simulink model "Roombaavancet_newnewnewnew"  (R2018b)
settings: Solver=FixedStepDiscrete  StartTime=0.0  StopTime=inf  FixedStep=0.1  RelTol=1e-3
InitFcn:
  | iRobotControl_switchyard('setup_localPCclock');iRobotControl_switchyard('setup_StarGazer_landmark_offset_table')
undefined symbols (not defined in the file or in its folder): iRobotControl_switchyard, none, Rec, SDTV, videoinput
libraries: visiontransforms x2, visionconversions x1, visiontextngfix x1, visionanalysis x1, visionstatistics x1, imaqlib x1, realtime_pacer_lib x1, visionsinks x1
CloseFcn:
  | iRobotControl_switchyard close_iRobotControl
settings Model: Creator=sksu  LastModifiedBy=chada
settings SolverCC: PositivePriorityOrder=on
settings DataIOCC: LimitDataPoints=on  SaveFormat=Array  SignalLoggingSaveFormat=ModelDataLogs
settings OptimizationCC: EnhancedBackFolding=on  PassReuseOutputArgsAs=Individual arguments  ExpressionDepthLimit=2147483647  MaxStackSize=64  OptimizeBlockOrder=speed  DifferentSizesBufferReuse=on  OptimizationCustomize=off
settings DebuggingCC: UnderspecifiedInitializationDetection=Classic  MergeDetectMultiDrivingBlocksExec=none  SolverPrmCheckMsg=warning  ParameterTunabilityLossMsg=error  FcnCallInpInsideContextMsg=warning  AllowSymbolicDim=off  StateNameClashWarn=warning  SFUnexpectedBacktrackingDiag=warning  SFNoUnconditionalDefaultTransitionDiag=warning  SFExecutionAtInitializationDiag=none
settings HardwareCC: ProdBitPerPointer=32  ProdBitPerSizeT=32  ProdBitPerPtrDiffT=32  ProdLargestAtomicInteger=Long  ProdLargestAtomicFloat=Double  ProdWordSize=32  ProdHWDeviceType=ARM Compatible->ARM Cortex
settings ModelReferenceCC: PropagateSignalLabelsOutOfModel=off
settings SFSimCC: SimUseLocalCustomCode=off  MATLABDynamicMemAlloc=off
settings RTWCC: SystemTargetFile=ert.tlc  HardwareBoard=Raspberry Pi  TLCOptions="-aInlineSetEventsForThisBaseRateFcn=TLC_FALSE -aSuppressMultiTaskScheduler=TLC_FALSE  -aRateBasedStepFcn=0"  TemplateMakefile=ert_default_tmf  GenerateReport=on  RTWUseLocalCustomCode=off  Toolchain=GNU GCC Raspberry Pi  BuildConfiguration=Faster Runs  IncludeHyperlinkInReport=on  LaunchReport=on  GenerateTraceInfo=on  GenerateTraceReport=on  GenerateTraceReportSl=on  GenerateTraceReportSf=on  GenerateTraceReportEml=on
settings CodeAppCC: ForceParamTrailComments=on  IgnoreCustomStorageClasses=off  OperatorAnnotations=on  SimulinkDataObjDesc=on  SFDataObjDesc=on  InsertBlockDesc=on
settings ERTTargetCC: SupportVariableSizeSignals=on
settings ConfigComp: CovMetricSettings=dw  CovHtmlReporting=on  CovSaveCumulativeToWorkspaceVar=on  CovSaveSingleToWorkspaceVar=on  CovExternalEMLEnable=off

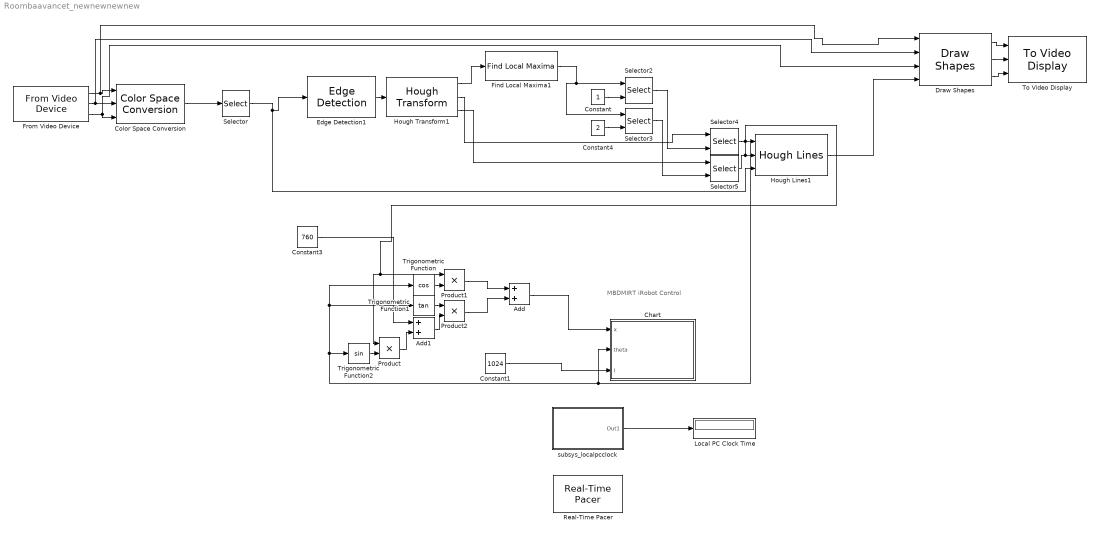
== system Roombaavancet_newnewnewnew ==
  note: MBDMIRT iRobot Control
  Add : Sum
  Add1 : Sum
  Chart : Stateflow chart  TreatAsAtomicUnit=on
  Color Space Conversion : visionconversions/Color Space  Conversion  conversion=Obsolete  conversionActive=R'G'B' to intensity  wp_str=D65  rec=Rec. 601 (SDTV)  sys=1125/60/2:1  imagePorts=Separate color signals
      settings: SourceProductName=Computer Vision System Toolbox
  Constant : Constant
  Constant1 : Constant  Value=1024
  Constant3 : Constant  Value=760
  Constant4 : Constant  Value=2
  Draw Shapes : visiontextngfix/Draw Shapes  shape=Lines  fill=off  lineWidth=10  fillClrSource=Specify via dialog  display=User-specified value  intensity=200  color=[000 000 255]  opacity=0.6  viewport=Entire image  antialiasing=off  inType=Obsolete  imagePorts=Separate color signals  prodOutputMode=Binary point scaling  prodOutputWordLength=32  prodOutputFracLength=14  memoryMode=Specify word length  memoryWordLength=16  memoryFracLength=14  roundingMode=Floor  overflowMode=off
      settings: SourceProductName=Computer Vision System Toolbox
  Edge Detection1 : visionanalysis/Edge Detection  method=Sobel  outputType=Binary image  userDefinedThreshold=off  thresholdSource=Input port  threshold=20  thresholdTuning=4  edgeThinning=off  threshold_canny=[0.25 0.60]  autoPercent=70  sigma=1  roundingMode=Floor  overflowMode=off  prodOutputMode=Binary point scaling  prodOutputWordLength=32  prodOutputFracLength=8  prodOutputSlope=2^-8  accumSlope=2^-8  outputSlope=2^-4
      settings: SourceProductName=Computer Vision System Toolbox  SourceProductBaseCode=VP
  Find Local Maxima1 : visionstatistics/Find Local Maxima  num_peaks=1  nhood_size=[801 201]  src_thresh=Obsolete9b  src_thresh_inuse=Specify via dialog  threshold=10  inputIsHough=on  dt_peak=uint32  isOutVarDim=on  dt_count=uint32
      settings: SourceProductName=Computer Vision System Toolbox  SourceProductBaseCode=VP
  From Video Device : imaqlib/From Video Device  DeviceMenu=(none)  Device=winvideo 1 (Webcam C170)  ObjConstructor=videoinput('winvideo', 1)  VideoFormatMenu=(none)  VideoFormat=MJPG_1024x768  VideoSource=input1  ROIPosition=[0 0 768 1024]  EnableHWTrigger=off  TriggerConfiguration=none/none  SampleTime=0.1  OutputPortsMode=Separate color signals  DataType=single  CanDoHWTrigger=no  ReturnedColorSpace=rgb  BlockHandle=146.0004  ROIWidth=1024  ROIHeight=768  ROIColumn=0  ROIRow=0  EngXMLPath=C:\Program Files\MATLAB\R2018b\toolbox\imaq\imaq\private  DevXMLPath=C:\ProgramData\MATLAB\SupportPackages\R2018b\toolbox\imaq\supportpackages\genericvideo\adaptor\win64  EngLibPath=C:\Program Files\MATLAB\R2018b\toolbox\imaq\imaqblks\imaqmex\win64  ColorSpace=rgb  BayerSensorAlignment=grbg
      settings: SourceProductName=Image Acquisition Toolbox
  Hough Lines1 : visiontransforms/Hough Lines  sineCompMethod=Trigonometric function  thetaRes=pi/180  firstCoeffMode=Specify word length  firstCoeffWordLength=16  firstCoeffFracLength=15  prodOutputMode=Binary point scaling  prodOutputWordLength=32  prodOutputFracLength=16  roundingMode=Nearest  overflowMode=on
      settings: SourceProductName=Computer Vision System Toolbox  SourceProductBaseCode=VP
  Hough Transform1 : visiontransforms/Hough Transform  theta_res=pi/360  rho_res=1  out_theta_rho=on  outdtmode=double  roundingMode=Nearest  overflowMode=on  firstCoeffMode=Binary point scaling  firstCoeffWordLength=16  firstCoeffFracLength=14  firstCoeffSlope=2^-14  secondCoeffMode=Binary point scaling  secondCoeffWordLength=32  secondCoeffFracLength=16  secondCoeffSlope=2^-16  prodOutputMode=Binary point scaling  prodOutputWordLength=32  prodOutputFracLength=20  prodOutputSlope=2^-20  accumMode=Binary point scaling  accumWordLength=32  accumFracLength=20  accumSlope=2^-20  outputMode=Binary point scaling  outputWordLength=16  outputFracLength=0  outputSlope=2^0  memoryMode=Binary point scaling  memoryWordLength=32  memoryFracLength=16  memorySlope=2^-16
      settings: SourceProductName=Computer Vision System Toolbox  SourceProductBaseCode=VP
  Local PC Clock Time : Display
  Product : Product
  Product1 : Product
  Product2 : Product
  Real-Time Pacer : realtime_pacer_lib/Real-Time Pacer  simTimePerRealTime=1000
  Selector : Selector  NumberOfDimensions=2  InputPortWidth=3  IndexOptions=Starting index (dialog),Select all  Indices=[1],1  OutputSizes=[760],1
  Selector2 : Selector  InputPortWidth=2  IndexOptions=Index vector (port)  Indices=1  OutputSizes=1
  Selector3 : Selector  InputPortWidth=2  IndexOptions=Index vector (port)  Indices=0  OutputSizes=1
  Selector4 : Selector  InputPortWidth=360  IndexOptions=Index vector (port)  Indices=[1 3]  OutputSizes=1
  Selector5 : Selector  InputPortWidth=2549  IndexOptions=Index vector (port)  Indices=[1 3]  OutputSizes=1
  To Video Display : visionsinks/To Video Display  windowSizeMode=Normal  openAtMdlStart=on  fullScreen=off  videoWindowX=0  videoWindowY=22  saveWindowSize=off  videoWindowWidth=1440  videoWindowHeight=838  inputColorFormat=RGB  inputType=Obsolete  imagePorts=Separate color signals  OutputDevice=On-screen video monitor  dataOrg=Column-major  isWindowOpen=off
      settings: SourceProductName=Computer Vision System Toolbox
  Trigonometric Function : Trigonometry  Operator=cos
  Trigonometric Function1 : Trigonometry  Operator=tan
  Trigonometric Function2 : Trigonometry
  subsys_localpcclock : Subsystem
      mask Display: fprintf('Elapsed Local PC\nClock')
  wires:
  subsys_localpcclock/1(Out1) -> Local PC Clock Time/1
  Trigonometric Function/1 -> Product1/2
  Product1/1 -> Add/1
  Product2/1 -> Add/2
  Trigonometric Function1/1 -> Product2/1
  Add1/1 -> Product2/2
  Product/1 -> Add1/2
  Trigonometric Function2/1 -> Product/2
  Selector4/1 -> Chart/2(theta), Trigonometric Function1/1, Trigonometric Function/1, Trigonometric Function2/1, Hough Lines1/1
  Selector5/1 -> Product/1, Product1/1, Hough Lines1/2
  Constant3/1 -> Add1/1
  Constant4/1 -> Selector3/2
  Hough Transform1/3 -> Selector5/1
  Hough Transform1/2 -> Selector4/1
  Selector2/1 -> Selector4/2
  Selector3/1 -> Selector5/2
  Edge Detection1/1 -> Hough Transform1/1
  Constant/1 -> Selector2/2
  Find Local Maxima1/1 -> Selector3/1, Selector2/1
  Hough Transform1/1 -> Find Local Maxima1/1
  From Video Device/2 -> Color Space Conversion/2, Draw Shapes/2
  From Video Device/1 -> Draw Shapes/1, Color Space Conversion/1
  From Video Device/3 -> Color Space Conversion/3, Draw Shapes/3
  Hough Lines1/1 -> Draw Shapes/4
  Draw Shapes/2 -> To Video Display/2
  Draw Shapes/1 -> To Video Display/1
  Draw Shapes/3 -> To Video Display/3
  Color Space Conversion/1 -> Selector/1
  Selector/1 -> Hough Lines1/3, Edge Detection1/1
  Add/1 -> Chart/1(x)
  Constant1/1 -> Chart/3(l)

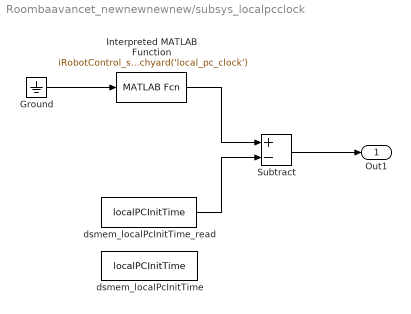
== system Roombaavancet_newnewnewnew/subsys_localpcclock ==
  Ground : Ground
  Interpreted MATLAB Function : MATLABFcn  MATLABFcn=iRobotControl_switchyard('local_pc_clock')  OutputSignalType=real
  Subtract : Sum  Inputs=+-
  dsmem_localPcInitTime : DataStoreMemory  DataStoreName=localPCInitTime  WriteAfterWriteMsg=warning  WriteAfterReadMsg=warning  InitialValue=2390464.087  ShowAdditionalParam=off  OutDataTypeStr=double
  dsmem_localPcInitTime_read : DataStoreRead  DataStoreName=localPCInitTime  SampleTime=1
  Out1 : Outport
  wires:
  Ground/1 -> Interpreted MATLAB Function/1
  Interpreted MATLAB Function/1 -> Subtract/1
  dsmem_localPcInitTime_read/1 -> Subtract/2
  Subtract/1 -> Out1/1

== stateflow chart Roombaavancet_newnewnewnew/Chart ==
  settings: updateMethod=DISCRETE  sampleTime=1
  state AngleR = AngleSensorRoomba(serObjNum) [function]
    (default) -> (junction 640) : { AngleR = ml('AngleSensorRoomba(iRobot_%d)', serObjNum); }
  state clk = LocalPCClock [function]
    (default) -> (junction 1924) : {clk = ml.iRobotControl_switchyard('local_pc_clock');}
  state state = CliffRightSensorRoomba(serObjNum) [function]
    (default) -> (junction 756) : { state = ml('CliffRightSensorRoomba(iRobot_%d)', serObjNum); }
  state [Charge, Capacity, Percent] = BatteryChargeReaderRoomba(serObjNum) [function]
    (default) -> (junction 665) : {
        | /* Reset container for battery status */
        | ml('iRobot_%d_BattCharSensor(1:3)=0;', serObjNum);
        |
        | /* Read battery status */
        | ml('[iRobot_%d_BattCharSensor(1), iRobot_%d_BattCharSensor(2), iRobot_%d_BattCharSensor(3)]=BatteryChargeReaderRoomba(iRobot_%d);',...
        |       serObjNum, serObjNum, serObjNum, serObjNum);
        |
        |
        | BattCharSensor=ml('iRobot_%d_BattCharSensor', serObjNum);
        |
        | Charge=BattCharSensor[0];
        | Capacity=BattCharSensor[1];
        | Percent=BattCharSensor[2];
        | }
  state strg = CliffRightSignalStrengthRoomba(serObjNum) [function]
    (default) -> (junction 761) : { strg = ml('CliffRightSignalStrengthRoomba(iRobot_%d)', serObjNum); }
  state BeepRoomba(serObjNum) [function]
    (default) -> (junction 686) : { ml('BeepRoomba(iRobot_%d)', serObjNum); }
  state iRobot_Test
    state INIT
      en: irobotID=1;
      serObjNum=RoombaInit(irobotID)
    state DEPLACEMENT
      du:
      [Dock, Clean] = ButtonsSensorRoomba(serObjNum);
      state STOP
        en: SetFwdVelAngVelCreate(serObjNum, 0, 0);
        SetLEDsRoomba(serObjNum, 0, 10, 100);
        SetBrushRoomba(serObjNum, 0);
      state Fwd_Bwd
        state Robot_avance_vitesseConstante
          en:
          SetFwdVelAngVelCreate(serObjNum, 0.05, 0);
          seenClk=LocalPCClock();
          du:
          currClk=LocalPCClock();
        state corrige
          en:
          SetFwdVelAngVelCreate(serObjNum,0.05,- 0.1*(theta)/(abs(theta)));
        (default) -> Robot_avance_vitesseConstante
        corrige -> Robot_avance_vitesseConstante : [abs(x-(l/2))<1 && abs(theta)<0.2]
        Robot_avance_vitesseConstante -> corrige : [abs(x-(l/2))>1 || abs(theta)>0.2]
      (default) -> STOP
      Fwd_Bwd -> STOP : [Dock]
      STOP -> Fwd_Bwd : [Clean]
    note: ?
    (default) -> INIT
    INIT -> DEPLACEMENT
  state [BumpRight, BumpLeft, WheDropRight, WheDropLeft, ... [function]
    WheDropCaster, BumpFront] = BumpsWheelDropsSensorsRoomba(serObjNum)
    (default) -> (junction 455) : {
        | /* Reset container for bump and wheel sensors */
        | ml('iRobot_%d_BmpWhlSensor(1:6)=0;', serObjNum);
        |
        | /* Read bump and wheel sensors */
        | ml('[iRobot_%d_BmpWhlSensor(1), iRobot_%d_BmpWhlSensor(2), iRobot_%d_BmpWhlSensor(3), iRobot_%d_BmpWhlSensor(4), iRobot_%d_BmpWhlSensor(5), iRobot_%d_BmpWhlSensor(6)]=BumpsWheelDropsSensorsRoomba(iRobot_%d);',...
        |       serObjNum, serObjNum, serObjNum, serObjNum, serObjNum, serObjNum, serObjNum);
        |
        |
        | BmpWhlSensor = ml('iRobot_%d_BmpWhlSensor', serObjNum);
        |
        | BumpRight=BmpWhlSensor[0];
        | BumpLeft=BmpWhlSensor[1];
        | WheDropRight=BmpWhlSensor[2];
        | WheDropLeft=BmpWhlSensor[3];
        | WheDropCaster=BmpWhlSensor[4];
        | BumpFront=BmpWhlSensor[5];
        | }
  state Current = CurrentTesterRoomba(serObjNum) [function]
    (default) -> (junction 766) : { Current = ml('CurrentTesterRoomba(iRobot_%d)', serObjNum); }
  state [ButtonAdv, ButtonPlay] = ButtonsSensorRoomba(serObjNum) [function]
    (default) -> (junction 694) : {
        | /* Reset container for buttons seonsor */
        | ml('iRobot_%d_ButtSensor(1:2)=0;', serObjNum);
        |
        | /* Read battery status */
        | ml('[iRobot_%d_ButtSensor(1), iRobot_%d_ButtSensor(2)]=ButtonsSensorRoomba(iRobot_%d);',...
        |       serObjNum, serObjNum, serObjNum);
        |
        |
        | ButtSensor=ml('iRobot_%d_ButtSensor', serObjNum);
        |
        | ButtonAdv=ButtSensor[0];
        | ButtonPlay=ButtSensor[1];
        | }
  state Distance = DistanceSensorRoomba(serObjNum) [function]
    (default) -> (junction 801) : { Distance = ml('DistanceSensorRoomba(iRobot_%d)', serObjNum); }
  state state = CliffFrontLeftSensorRoomba(serObjNum) [function]
    (default) -> (junction 718) : { state = ml('CliffFrontLeftSensorRoomba(iRobot_%d)', serObjNum); }
  state serObjNum = RoombaInit(irobotID) [function]
    (default) -> (junction 574) : /* Check if expected variable exists*/
        | { flag_exist=ml('exist(''iRobot_%d'',''var'')', irobotID); }
    (junction 574) -> (junction 575) [order 1] : [ flag_exist==true ]
    (junction 575) -> (junction 580) : /* Check if the expected variable is a serial object */
        | { flag_serport=ml('isa(iRobot_%d, ''serial'')', irobotID); }
    (junction 574) -> (junction 578) [order 2]
    (junction 580) -> (junction 576) [order 1] : [ flag_serport==true ]
    (junction 580) -> (junction 577) [order 2]
    (junction 576) -> (junction 581) : { serObjNum=irobotID; }
    (junction 577) -> (junction 578)
    (junction 578) -> (junction 2272) : { ml.error('iRobot_%d is not initialized.', irobotID); }
  state strg = CliffFrontLeftSignalStrengthRoomba(serObjNum) [function]
    (default) -> (junction 729) : { strg = ml('CliffFrontLeftSignalStrengthRoomba(iRobot_%d)', serObjNum); }
  state SetDriveWheelsCreate(serObjNum, rightWheelVel, leftWheelVel) [function]
    (default) -> (junction 809) : { ml('SetDriveWheelsCreate(iRobot_%d, %f, %f)', serObjNum, rightWheelVel, leftWheelVel); }
  state state = CliffFrontRightSensorRoomba(serObjNum) [function]
    (default) -> (junction 736) : { state = ml('CliffFrontRightSensorRoomba(iRobot_%d)', serObjNum); }
  state SetFwdVelAngVelCreate(serObjNum, FwdVel, AngVel) [function]
    (default) -> (junction 65) : { ml('SetFwdVelAngVelCreate(iRobot_%d, %f, %f)', serObjNum, FwdVel, AngVel); }
  state SetBrushRoomba(serObjNum, Brushes) [function]
    (default) -> (junction 3475) : { ml('SetBrushRoomba(iRobot_%d, %f)', serObjNum, Brushes); }
  state SetFwdVelRadiusRoomba(serObjNum, FwdVel, Radius) [function]
    (default) -> (junction 816) : { ml('SetFwdVelRadiusRoomba(iRobot_%d, %f, %f)', serObjNum, FwdVel, Radius); }
  state strg = CliffFrontRightSignalStrengthRoomba(serObjNum) [function]
    (default) -> (junction 741) : { strg = ml('CliffFrontRightSignalStrengthRoomba(iRobot_%d)', serObjNum); }
  state SetLCDRoomba(serObjNum, D3,D2,D1,D0) [function]
    (default) -> (junction 3466) : { ml('SetLCDRoomba(iRobot_%d, %f, %f, %f, %f)', serObjNum, D3, D2, D1, D0); }
  state state = CliffLeftSensorRoomba(serObjNum) [function]
    (default) -> (junction 746) : { state = ml('CliffLeftSensorRoomba(iRobot_%d)', serObjNum); }
  state SetLEDsRoomba(serObjNum, LED,Color, Intensity) [function]
    (default) -> (junction 823) : { ml('SetLEDsRoomba(iRobot_%d, %f, %f, %f)', serObjNum, LED, Color, Intensity); }
  state strg = CliffLeftSignalStrengthRoomba(serObjNum) [function]
    (default) -> (junction 751) : { strg = ml('CliffLeftSignalStrengthRoomba(iRobot_%d)', serObjNum); }
  state travelDist(serObjNum, speed, distance) [function]
    (default) -> (junction 294) : { ml('travelDist(iRobot_%d, %f, %f)', serObjNum, speed, distance); }
  state turnAngle(serObjNum, speed, angle) [function]
    (default) -> (junction 335) : { ml('turnAngle(iRobot_%d, %f, %f)', serObjNum, speed, angle); }
  (default) -> iRobot_Test
  data: serObjNum function_input int16; AngleR function_output double; clk function_output double; serObjNum function_input int16; state function_output double; Charge function_output double; Capacity function_output double; Percent function_output double; serObjNum function_input int16; BattCharSensor temporary double size=1,3; serObjNum function_input int16; strg function_output double; serObjNum function_input int16; serObjNum local double; bR local double; bL local double; wR local double; wL local double; wCst local double; bF local double; ang_turned local double; irobotID local double; pi parameter double; currClk local double; seenClk local double; xold local double; BumpRight function_output double; BumpLeft function_output double; WheDropRight function_output double; WheDropLeft function_output double; WheDropCaster function_output double; serObjNum function_input int16; BumpFront function_output double; BmpWhlSensor temporary double size=1,6; serObjNum function_input int16; Current function_output double; ButtonAdv function_output double; ButtonPlay function_output double; serObjNum function_input int16; ButtSensor temporary double size=1,2; Distance function_output double; serObjNum function_input int16; serObjNum function_input int16; state function_output double; irobotID function_input int16; serObjNum function_output int16; flag_serport temporary boolean; flag_exist temporary boolean; serObjNum function_input int16; strg function_output double; serObjNum function_input int16; rightWheelVel function_input double; leftWheelVel function_input double; serObjNum function_input int16; state function_output double; serObjNum function_input int16; FwdVel function_input double; AngVel function_input double; serObjNum function_input int16; Brushes function_input double; serObjNum function_input int16; FwdVel function_input double; Radius function_input double; serObjNum function_input int16; strg function_output double; serObjNum function_input int16; D3 function_input double; D2 function_input double; D1 function_input double; D0 function_input double; serObjNum function_input int16; state function_output double; serObjNum function_input int16; LED function_input double; Color function_input double; Intensity function_input double; serObjNum function_input int16; strg function_output double; serObjNum function_input int16; speed function_input double; distance function_input double; serObjNum function_input int16; speed function_input double; angle function_input double; cf_FL local double; cf_FR local double; fwdVel local double; irobotID local double; radi_L local double; radi_S local double; serObjNum local double; BumpLeft local double; BumpRight local double; WheDropCaster local double; WheDropLeft local double; WheDropRight local double; BumpFront local double; Dock local double; Clean local double; x input double; theta input double; l input double
  events: ButtonClean local FUNCTION_CALL_EVENT; ButtonDock local FUNCTION_CALL_EVENT
